simulink subsystem "CVT"  (R2020a)
settings: Solver=VariableStepAuto  StartTime=0.0  StopTime=10.0  RelTol=1e-3
libraries: fl_lib x10, nesl_utility x2, sdl_lib x1
settings Model: Creator=Tyler  LastModifiedBy=Tyler

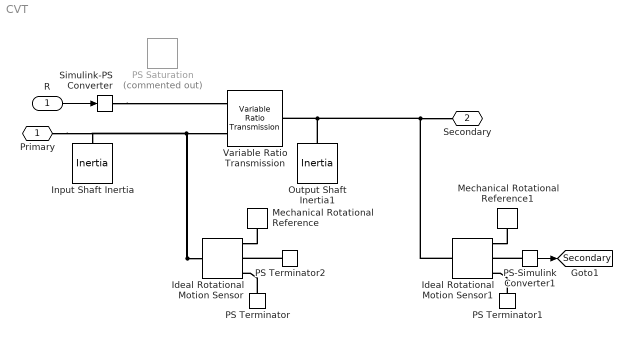
== system CVT ==
  R : Inport
  Ideal Rotational Motion Sensor : fl_lib/Mechanical/Mechanical Sensors/Ideal Rotational Motion Sensor  wrap_angle=simscape.enum.onoff.off  offset=0 rad
  Ideal Rotational Motion Sensor1 : fl_lib/Mechanical/Mechanical Sensors/Ideal Rotational Motion Sensor  wrap_angle=simscape.enum.onoff.off  offset=0 rad
  Input Shaft Inertia : fl_lib/Mechanical/Rotational Elements/Inertia  inertia=0.01 kg*m^2  w_specify=on  w_priority=Low  w=1700 rpm  w_nominal_specify=off  w_nominal_unit=rad/s  w_nominal_value=1  t_specify=off  t_priority=None  t=0 N*m  t_nominal_specify=off  t_nominal_unit=N*m  t_nominal_value=1
  Mechanical Rotational Reference : fl_lib/Mechanical/Rotational Elements/Mechanical Rotational Reference
  Mechanical Rotational Reference1 : fl_lib/Mechanical/Rotational Elements/Mechanical Rotational Reference
  Output Shaft Inertia1 : fl_lib/Mechanical/Rotational Elements/Inertia  inertia=0.01 kg*m^2  w_specify=off  w_priority=High  w=0 rad/s  w_nominal_specify=off  w_nominal_unit=rad/s  w_nominal_value=1  t_specify=off  t_priority=None  t=0 N*m  t_nominal_specify=off  t_nominal_unit=N*m  t_nominal_value=1
  PS Saturation : fl_lib/Physical Signals/Nonlinear Operators/PS Saturation  Commented=on  upper_limit=0.5  lower_limit=-0.5
      settings: SourceProductBaseCode=SS
  PS Terminator : fl_lib/Physical Signals/Sinks/PS Terminator
  PS Terminator1 : fl_lib/Physical Signals/Sinks/PS Terminator
  PS Terminator2 : fl_lib/Physical Signals/Sinks/PS Terminator
  PS-Simulink Converter1 : nesl_utility/PS-Simulink Converter  PhysicalDomain=network_engine_domain  SubClassName=ps_output  LeftPortType=input  RightPortType=output  PseudoPeriodic=off  Frequencies=[]  Unit=rpm  AffineConversion=off
  Simulink-PS Converter : nesl_utility/Simulink-PS Converter  PhysicalDomain=network_engine_domain  SubClassName=ps_input  LeftPortType=input  RightPortType=output  PseudoPeriodic=off  Frequencies=[]  NoiseDistribution=none  NoiseParameters=[]  Unit=1  AffineConversion=off  FilteringAndDerivatives=provide  SimscapeFilterOrder=1  InputFilterTimeConstant=0.001  UdotUserProvided=0
  Variable Ratio Transmission : sdl_lib/Couplings & Drives/Variable Ratio Transmission  rotation_direction=1  kp=3e5 N*m/rad  kv=0.05 N*m/(rad/s)  initial_torque=0 N*m  losses_model=1  efficiency=0.8  mu_visc=[0, 0] N*m/(rad/s)  w_thr=0.01 rad/s  R_specify=off  R_priority=None  R=1  R_nominal_specify=off  R_nominal_unit=1  R_nominal_value=1
      settings: SourceProductBaseCode=LD  InternalSimscapePortConfiguration="{\"Bottom\":[],\"Left\":[{\"id\":\"ratio\",\"label\":\"r\",\"type\":\"input\"},{\"id\":\"B\",\"label\":\"B\",\"type\":\"foundation.mechanical.rotational.rotational\"}],\"Right\":[{\"id\":\"F\",\"label\":\"F\",\"type\":\"foundation.mechanical.rotational.rotational\"}],\"Top\":[]}"
  Primary : PMIOPort  Side=Left
  Secondary : PMIOPort  Port=2  Side=Right
  tag scope: Secondary=global
  wires:
  PS-Simulink Converter1/1 -> [Secondary]
  R/1 -> Simulink-PS Converter/1
  connections:
  Ideal Rotational Motion Sensor/LConn1 -- Primary/RConn1 -- Input Shaft Inertia/LConn1 -- Variable Ratio Transmission/LConn2
  Ideal Rotational Motion Sensor1/LConn1 -- Output Shaft Inertia1/LConn1 -- Variable Ratio Transmission/RConn1 -- Secondary/RConn1
  PS Terminator/LConn1 -- Ideal Rotational Motion Sensor/RConn3
  Ideal Rotational Motion Sensor/RConn1 -- Mechanical Rotational Reference/LConn1
  PS Terminator2/LConn1 -- Ideal Rotational Motion Sensor/RConn2
  PS-Simulink Converter1/LConn1 -- Ideal Rotational Motion Sensor1/RConn2
  Ideal Rotational Motion Sensor1/RConn1 -- Mechanical Rotational Reference1/LConn1
  PS Terminator1/LConn1 -- Ideal Rotational Motion Sensor1/RConn3
  Simulink-PS Converter/RConn1 -- Variable Ratio Transmission/LConn1
